simulink model "floating_pend_2D_to_workspace"  (R2019b)
settings: Solver=FixedStepAuto  StartTime=0.0  StopTime=100  FixedStep=0.01  RelTol=1e-3
settings Model: Creator=Murray  LastModifiedBy=Murray

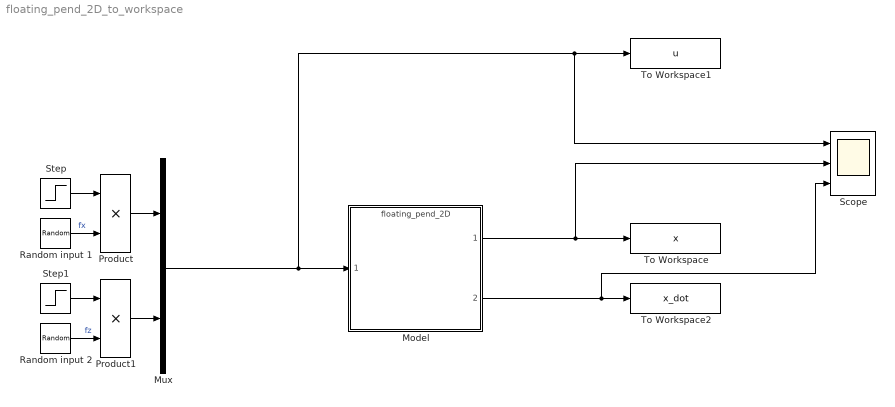
== system floating_pend_2D_to_workspace ==
  Model : ModelReference  ModelNameDialog=floating_pend_2D.slx  SimulationMode=Normal  ModelReferenceVersion=1.24
  Mux : Mux  Inputs=2
  Product : Product
  Product1 : Product
  Random input 1 : RandomNumber  Variance=25  Seed=2  SampleTime=5
  Random input 2 : RandomNumber  Mean=6*9.81  Variance=25  Seed=1  SampleTime=5
  Scope : Scope  NumInputPorts=3
  Step : Step  Before=1  SampleTime=0
  Step1 : Step  Before=1  SampleTime=0
  To Workspace : ToWorkspace  VariableName=x  SaveFormat=Timeseries  SampleTime=-1
  To Workspace1 : ToWorkspace  VariableName=u  SaveFormat=Timeseries  SampleTime=-1
  To Workspace2 : ToWorkspace  VariableName=x_dot  SaveFormat=Timeseries  SampleTime=-1
  wires:
  Model/1 -> Scope/2, To Workspace/1
  Mux/1 -> Scope/1, To Workspace1/1, Model/1
  Model/2 -> Scope/3, To Workspace2/1
  Step/1 -> Product/1
  Random input 1/1 -> Product/2  "fx"
  Product/1 -> Mux/1
  Step1/1 -> Product1/1
  Product1/1 -> Mux/2
  Random input 2/1 -> Product1/2  "fz"
